simulink library "INP_DMP"  (R2024b)
settings: Solver=VariableStepAuto  StartTime=0.0  StopTime=10.0  RelTol=1e-3
libraries: INP_DMP_ManOver x1, INP_DMP_Prep x1
settings Model: Creator=blatak  LastModifiedBy=jmbsp
settings ModelReferenceCC: EnableRefExpFcnMdlSchedulingChecks=on
settings RTWCC: GPUComputeCapability=3.5

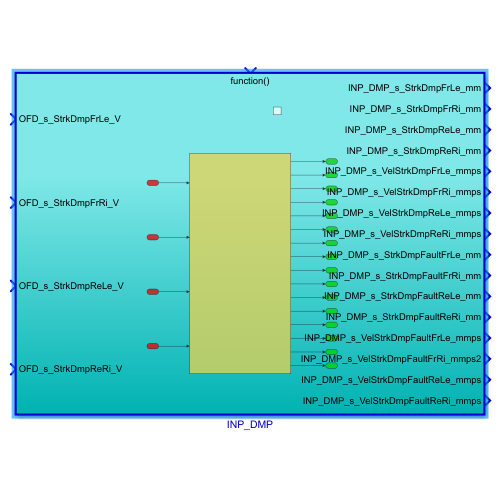
[thumbnail: Simulink's stored preview of the top-level diagram]
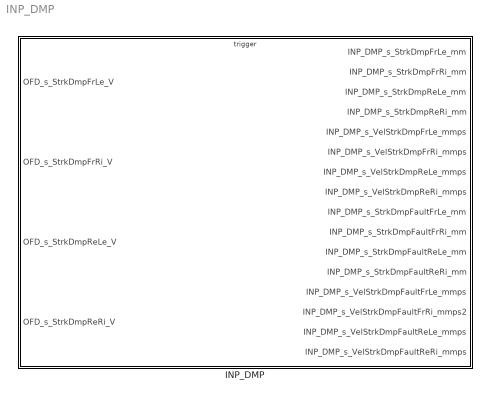
== system INP_DMP ==
  INP_DMP : Subsystem  TreatAsAtomicUnit=on

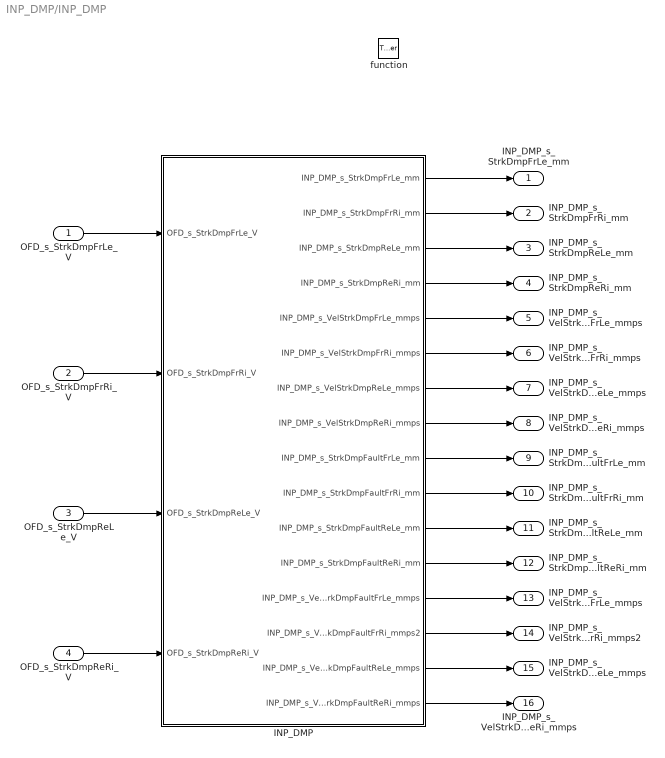
== system INP_DMP/INP_DMP ==
  OFD_s_StrkDmpFrLe_V : Inport
  OFD_s_StrkDmpFrRi_V : Inport  Port=2
  OFD_s_StrkDmpReLe_V : Inport  Port=3
  OFD_s_StrkDmpReRi_V : Inport  Port=4
  function : TriggerPort  TriggerType=function-call  VariantControl=(inherit)
  INP_DMP : Subsystem
  INP_DMP_s_StrkDmpFrLe_mm : Outport
  INP_DMP_s_StrkDmpFrRi_mm : Outport  Port=2
  INP_DMP_s_StrkDmpReLe_mm : Outport  Port=3
  INP_DMP_s_StrkDmpReRi_mm : Outport  Port=4
  INP_DMP_s_VelStrkDmpFrLe_mmps : Outport  Port=5
  INP_DMP_s_VelStrkDmpFrRi_mmps : Outport  Port=6
  INP_DMP_s_VelStrkDmpReLe_mmps : Outport  Port=7
  INP_DMP_s_VelStrkDmpReRi_mmps : Outport  Port=8
  INP_DMP_s_StrkDmpFaultFrLe_mm : Outport  Port=9
  INP_DMP_s_StrkDmpFaultFrRi_mm : Outport  Port=10
  INP_DMP_s_StrkDmpFaultReLe_mm : Outport  Port=11
  INP_DMP_s_StrkDmpFaultReRi_mm : Outport  Port=12
  INP_DMP_s_VelStrkDmpFaultFrLe_mmps : Outport  Port=13
  INP_DMP_s_VelStrkDmpFaultFrRi_mmps2 : Outport  Port=14
  INP_DMP_s_VelStrkDmpFaultReLe_mmps : Outport  Port=15
  INP_DMP_s_VelStrkDmpFaultReRi_mmps : Outport  Port=16
  wires:
  OFD_s_StrkDmpFrRi_V/1 -> INP_DMP/2(OFD_s_StrkDmpFrRi_V)
  OFD_s_StrkDmpFrLe_V/1 -> INP_DMP/1(OFD_s_StrkDmpFrLe_V)
  OFD_s_StrkDmpReLe_V/1 -> INP_DMP/3(OFD_s_StrkDmpReLe_V)
  OFD_s_StrkDmpReRi_V/1 -> INP_DMP/4(OFD_s_StrkDmpReRi_V)
  INP_DMP/1(INP_DMP_s_StrkDmpFrLe_mm) -> INP_DMP_s_StrkDmpFrLe_mm/1
  INP_DMP/2(INP_DMP_s_StrkDmpFrRi_mm) -> INP_DMP_s_StrkDmpFrRi_mm/1
  INP_DMP/3(INP_DMP_s_StrkDmpReLe_mm) -> INP_DMP_s_StrkDmpReLe_mm/1
  INP_DMP/4(INP_DMP_s_StrkDmpReRi_mm) -> INP_DMP_s_StrkDmpReRi_mm/1
  INP_DMP/5(INP_DMP_s_VelStrkDmpFrLe_mmps) -> INP_DMP_s_VelStrkDmpFrLe_mmps/1
  INP_DMP/6(INP_DMP_s_VelStrkDmpFrRi_mmps) -> INP_DMP_s_VelStrkDmpFrRi_mmps/1
  INP_DMP/7(INP_DMP_s_VelStrkDmpReLe_mmps) -> INP_DMP_s_VelStrkDmpReLe_mmps/1
  INP_DMP/8(INP_DMP_s_VelStrkDmpReRi_mmps) -> INP_DMP_s_VelStrkDmpReRi_mmps/1
  INP_DMP/9(INP_DMP_s_StrkDmpFaultFrLe_mm) -> INP_DMP_s_StrkDmpFaultFrLe_mm/1
  INP_DMP/10(INP_DMP_s_StrkDmpFaultFrRi_mm) -> INP_DMP_s_StrkDmpFaultFrRi_mm/1
  INP_DMP/11(INP_DMP_s_StrkDmpFaultReLe_mm) -> INP_DMP_s_StrkDmpFaultReLe_mm/1
  INP_DMP/12(INP_DMP_s_StrkDmpFaultReRi_mm) -> INP_DMP_s_StrkDmpFaultReRi_mm/1
  INP_DMP/13(INP_DMP_s_VelStrkDmpFaultFrLe_mmps) -> INP_DMP_s_VelStrkDmpFaultFrLe_mmps/1
  INP_DMP/14(INP_DMP_s_VelStrkDmpFaultFrRi_mmps2) -> INP_DMP_s_VelStrkDmpFaultFrRi_mmps2/1
  INP_DMP/15(INP_DMP_s_VelStrkDmpFaultReLe_mmps) -> INP_DMP_s_VelStrkDmpFaultReLe_mmps/1
  INP_DMP/16(INP_DMP_s_VelStrkDmpFaultReRi_mmps) -> INP_DMP_s_VelStrkDmpFaultReRi_mmps/1

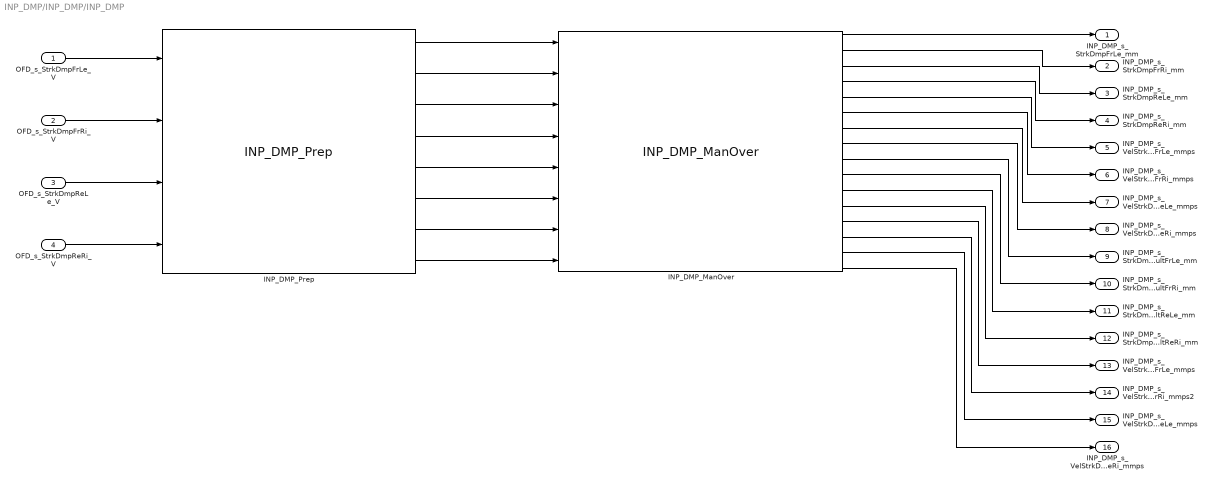
== system INP_DMP/INP_DMP/INP_DMP ==
  OFD_s_StrkDmpFrLe_V : Inport
  OFD_s_StrkDmpFrRi_V : Inport  Port=2
  OFD_s_StrkDmpReLe_V : Inport  Port=3
  OFD_s_StrkDmpReRi_V : Inport  Port=4
  INP_DMP_ManOver : INP_DMP_ManOver/INP_DMP_ManOver  SystemSampleTime=-1  VariantActivationTime=update diagram  AllowFlexibleInterface=on  Latency=0  AutoFrameSizeCalculation=off
  INP_DMP_Prep : INP_DMP_Prep/INP_DMP_Prep  SystemSampleTime=-1  VariantActivationTime=update diagram  AllowFlexibleInterface=on  Latency=0  AutoFrameSizeCalculation=off
  INP_DMP_s_StrkDmpFrLe_mm : Outport
  INP_DMP_s_StrkDmpFrRi_mm : Outport  Port=2
  INP_DMP_s_StrkDmpReLe_mm : Outport  Port=3
  INP_DMP_s_StrkDmpReRi_mm : Outport  Port=4
  INP_DMP_s_VelStrkDmpFrLe_mmps : Outport  Port=5
  INP_DMP_s_VelStrkDmpFrRi_mmps : Outport  Port=6
  INP_DMP_s_VelStrkDmpReLe_mmps : Outport  Port=7
  INP_DMP_s_VelStrkDmpReRi_mmps : Outport  Port=8
  INP_DMP_s_StrkDmpFaultFrLe_mm : Outport  Port=9
  INP_DMP_s_StrkDmpFaultFrRi_mm : Outport  Port=10
  INP_DMP_s_StrkDmpFaultReLe_mm : Outport  Port=11
  INP_DMP_s_StrkDmpFaultReRi_mm : Outport  Port=12
  INP_DMP_s_VelStrkDmpFaultFrLe_mmps : Outport  Port=13
  INP_DMP_s_VelStrkDmpFaultFrRi_mmps2 : Outport  Port=14
  INP_DMP_s_VelStrkDmpFaultReLe_mmps : Outport  Port=15
  INP_DMP_s_VelStrkDmpFaultReRi_mmps : Outport  Port=16
  wires:
  OFD_s_StrkDmpFrLe_V/1 -> INP_DMP_Prep/1
  OFD_s_StrkDmpFrRi_V/1 -> INP_DMP_Prep/2
  OFD_s_StrkDmpReLe_V/1 -> INP_DMP_Prep/3
  OFD_s_StrkDmpReRi_V/1 -> INP_DMP_Prep/4
  INP_DMP_Prep/1 -> INP_DMP_ManOver/1
  INP_DMP_Prep/2 -> INP_DMP_ManOver/2
  INP_DMP_Prep/3 -> INP_DMP_ManOver/3
  INP_DMP_Prep/4 -> INP_DMP_ManOver/4
  INP_DMP_Prep/5 -> INP_DMP_ManOver/5
  INP_DMP_Prep/6 -> INP_DMP_ManOver/6
  INP_DMP_Prep/7 -> INP_DMP_ManOver/7
  INP_DMP_Prep/8 -> INP_DMP_ManOver/8
  INP_DMP_ManOver/9 -> INP_DMP_s_StrkDmpFaultFrLe_mm/1
  INP_DMP_ManOver/10 -> INP_DMP_s_StrkDmpFaultFrRi_mm/1
  INP_DMP_ManOver/11 -> INP_DMP_s_StrkDmpFaultReLe_mm/1
  INP_DMP_ManOver/12 -> INP_DMP_s_StrkDmpFaultReRi_mm/1
  INP_DMP_ManOver/13 -> INP_DMP_s_VelStrkDmpFaultFrLe_mmps/1
  INP_DMP_ManOver/14 -> INP_DMP_s_VelStrkDmpFaultFrRi_mmps2/1
  INP_DMP_ManOver/15 -> INP_DMP_s_VelStrkDmpFaultReLe_mmps/1
  INP_DMP_ManOver/16 -> INP_DMP_s_VelStrkDmpFaultReRi_mmps/1
  INP_DMP_ManOver/1 -> INP_DMP_s_StrkDmpFrLe_mm/1
  INP_DMP_ManOver/2 -> INP_DMP_s_StrkDmpFrRi_mm/1
  INP_DMP_ManOver/3 -> INP_DMP_s_StrkDmpReLe_mm/1
  INP_DMP_ManOver/4 -> INP_DMP_s_StrkDmpReRi_mm/1
  INP_DMP_ManOver/8 -> INP_DMP_s_VelStrkDmpReRi_mmps/1
  INP_DMP_ManOver/7 -> INP_DMP_s_VelStrkDmpReLe_mmps/1
  INP_DMP_ManOver/6 -> INP_DMP_s_VelStrkDmpFrRi_mmps/1
  INP_DMP_ManOver/5 -> INP_DMP_s_VelStrkDmpFrLe_mmps/1
